simulink library "VAlib"  (Simulink 8.3)
settings: Solver=ode45  SolverMode=SingleTasking  StartTime=0.0  StopTime=10.0  RelTol=1e-3
undefined symbols (not defined in the file): automatic
libraries: VAlib x3, simulink x1
settings Model: Creator=aisakov  LastModifiedBy=lexx

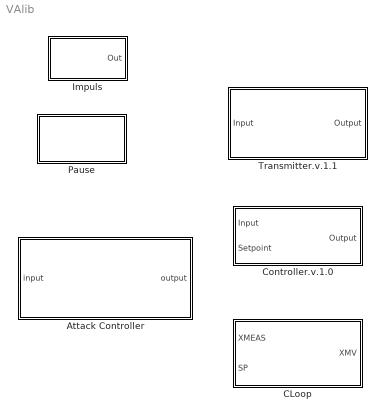
== system VAlib ==
  Attack Controller : Subsystem  mask(Attack controller){switch_mode=Integrity attack, atkMode=No attack, start=0, duration=1, Value=0, signalin=[], stime=-1, afterend=Holding final value}
      mask prompts: switch_mode "Attack Type:"; atkMode "Attack Mode:"; Value "Integrity Attack Value:"; signalin "Signal variable:"; stime "Sample time:"; afterend "Output after final:"
      mask help:
      | Attack controller block controls an attack on choosen variable on the specified time.
      | Attack types: DoS, Integrity and custom signal attack.
      | Modes: Step attack on specified time, Interval to specified time, Periodic and no attack.
      mask TypeOptions switch_mode: Integrity attack | DOS attack | Custom attack
      mask Callback switch_mode:
      | SM_MaskEnables = get_param(gcb, 'MaskEnables');
      | switch get_param(gcb, 'switch_mode')
      |     case 'Integrity attack'
      |         set_param([gcb,'/Switch value'], 'Value', '1');
      |         SM_MaskEnables{5} = 'on';
      |         SM_MaskEnables{6} = 'off';
      |         SM_MaskEnables{7} = 'off';
      |         SM_MaskEnables{8} = 'off';
      |     case 'DOS attack'
      |         set_param([gcb,'/Switch value'], 'Value', '3');
      |         SM_MaskEnables{5} = 'off';
      |         SM_MaskEnables{6} = 'off';
      |         SM_MaskEnables{7} = 'off';
      |         SM_MaskEnables{8} = 'off';
      |     case 'Custom attack'
      |         set_param([gcb,'/Switch value'], 'Value', '2');
      |         SM_MaskEnables{5} = 'off';
      |         SM_MaskEnables{6} = 'on';
      |         SM_MaskEnables{7} = 'on';
      |         SM_MaskEnables{8} = 'on';
      | end
      | set_param(gcb,'MaskEnables',SM_MaskEnables);
      | clear SM_MaskEnables;
      | 
      | % creat or remove block for custom attack
      | if strcmpi(get_param(gcb, 'switch_mode'), 'Custom attack') && ~exists_block([gcb '/SignalIn']) % creat block
      |     if exists_block([gcb, '/ReplaceBlock']);
      |         delete_line(gcb, 'ReplaceBlock/1', 'Multiport Switch/3');
      |         delete_block([gcb '/ReplaceBlock']);
      |     end
      | 
      |     add_block('built-in/FromWorkspace', [gcb '/SignalIn'], 'Position', [50 400 120 430]);
      |     add_line(gcb, 'SignalIn/1', 'Multiport Switch/3', 'autorouting', 'on');
      |     %set params
      |     set_param([gcb '/SignalIn'], 'SampleTime', '0');
      |     %set_param([gcb '/SignalIn'], 'VariableName', '[]');
      |     set_param([gcb '/SignalIn'], 'Interpolate', 'on');
      |     set_param([gcb '/SignalIn'], 'ZeroCross', 'off');
      |     %set_param([gcb '/' name], 'OutputAfterFinalValue', 'Setting to zero');
      |     %set_param([gcb '/' name], 'OutputAfterFinalValue', 'Cyclic repetition');
      |     %set_param([gcb '/' name], 'OutputAfterFinalValue', 'Extrapolation');
      |     %set_param([gcb '/' name], 'OutputAfterFinalValue', 'Holding final value');
      | 
      |     % forward signal parameters if set
      |     SW_signal = get_param(gcb, 'signalin');
      |     if strcmp(SW_signal, '[]') || strcmp(SW_signal, '') % signal not set
      |         set_param(gcb, 'signalin', '[]');
      |         set_param([gcb '/SignalIn'], 'VariableName', '[]');
      |         clear SW_signal;
      |         return;
      |     else    % signal set
      |         % check signal
      |         if ~exist(SW_signal)
      |             set_param(gcb, 'signalin', '[]');
      |             set_param([gcb '/SignalIn'], 'VariableName', '[]');
      |             warning(['Variable ' SW_signal ' not found.']);
      |             clear SW_signal;
      |             return;
      |         end
      |         SW_signal = evalin('base', SW_signal);
      |         if ~isvector(SW_signal)
      |             set_param(gcb, 'signalin', '');
      |             set_param([gcb '/SignalIn'], 'VariableName', '[]');
      |             warning(['Variable ' SW_signal ' must be a vector.']);
      |             clear SW_signal;
      |             return;
      |         end
      |         SW_stime = str2num(get_param(gcb, 'stime'));
      |         if isempty(SW_stime) || SW_stime < -1 || (SW_stime < 0 && SW_stime > -1)
      |             set_param(gcb, 'stime', '-1');
      |             SW_stime = -1;
      |             warning('Sample time must be a positive double or -1 for inherited value.');
      |         end
      | 
      |         if SW_stime == 0 || SW_stime == -1
      |             SW_stime = evalin('base', 'Ts_base');
      |         end
      | 
      |         SW_start = str2num(get_param(gcb, 'start'));
      |         SW_start = SW_stime * ceil(SW_start/SW_stime);
      |         signalstruct.time = SW_start:SW_stime:(SW_stime*(length(SW_signal) - 1) + SW_start);
      |         signalstruct.signals.values = SW_signal;
      | 
      | 		if strcmp(get_param(gcb, 'afterend'), 'Cyclic repetition')
      | 			SW_end = str2double(get_param(gcr, 'StopTime'));
      | 			while signalstruct.time(end) < SW_end
      | 				signalstruct.signals.values = [signalstruct.signals.values signalstruct.signals.values];
      | 				signalstruct.time = [signalstruct.time signalstruct.time+(signalstruct.time(end)-signalstruct.time(1))];
      | 			end
      | 		end
      | 
      | 		signalstruct.signals.values = signalstruct.signals.values(:);
      | 		signalstruct.time = signalstruct.time(:);
      |         %assignin('base', 'signalstruct', signalstruct)
      |         set_param([gcb '/SignalIn'], 'VariableName', 'signalstruct');
      |     end
      | 
      |     clear SW_signal;
      | 	clear SW_start;
      |     clear SW_stime;
      | 	clear SW_end;
      | elseif ~strcmpi(get_param(gcb, 'switch_mode'), 'Custom attack') && exists_block([gcb '/SignalIn']) % delete block
      |     delete_line(gcb, 'SignalIn/1', 'Multiport Switch/3');
      |     delete_block([gcb '/SignalIn']);
      |     % replace with constant value
      |     add_block(['built-in/Constant'], [gcb '/ReplaceBlock'], 'Position', [50 400 120 430]);
      |     add_line(gcb, ['ReplaceBlock/1'], 'Multiport Switch/3', 'autorouting', 'on');
      | end
      mask TypeOptions atkMode: Attack Type Controller/atkMode
      mask Callback atkMode:
      | AM_MaskEnables = get_param(gcb, 'MaskEnables');
      | switch get_param(gcb, 'atkMode');
      |     case 'No attack'
      |         AM_MaskEnables{3} = 'off';
      |         AM_MaskEnables{4} = 'off';
      |     case 'Step attack'
      |         AM_MaskEnables{3} = 'on';
      |         AM_MaskEnables{4} = 'off';
      |     otherwise
      |         AM_MaskEnables{3} = 'on';
      |         AM_MaskEnables{4} = 'on';
      | end
      | set_param(gcb, 'MaskEnables', AM_MaskEnables);
      | 
      | clear AM_MaskEnables;
      mask Callback start:
      | SS_start = get_param(gcb, 'start');
      | if strcmp(SS_start, '') % empty
      |     set_param(gcb, 'start', '0');
      |     SS_start = 0;
      | end
      | SS_start = str2num(SS_start);
      | if isempty(SS_start)
      |     set_param(gcb, 'start', '0');
      |     SS_start = 0;
      |     warning('Parameter value must be a nimeric value.');
      | end
      | 
      | % set to the subsystem
      | set_param([gcb '/Attack Type Controller'], 'start', get_param(gcb, 'start'));
      | 
      | % get correct signal parameters
      | if strcmpi(get_param(gcb, 'switch_mode'),'custom attack')
      |     if ~exists_block([gcb '/SignalIn'])
      |         clear SS_start;
      |         return
      |     end
      |     % forward signal parameters if set
      |     SS_signal = get_param(gcb, 'signalin');
      |     if strcmp(SS_signal, '[]') || strcmp(SS_signal, '') % signal not set
      |         clear SS_signal;
      |         clear SS_start;
      |         return;
      |     else    % signal set
      |         SS_signal = evalin('base', SS_signal);
      |         SS_stime = str2num(get_param(gcb, 'stime'));
      |         if isempty(SS_stime) || SS_stime < -1 || (SS_stime < 0 && SS_stime > -1)
      |             clear SS_signal;
      |             clear SS_start;
      |             set_param(gcb, 'stime', '-1');
      |             SS_stime = -1;
      |             warning('Sample time must be a positve double or -1 for inherited value.')
      |         end
      | 
      |         if SS_stime == 0 || SS_stime == -1
      |             SS_stime = evalin('base', 'Ts_base');
      |         end
      | 
      | 
      |         signalstruct.time = SS_start:SS_stime:(SS_stime*(length(SS_signal) - 1) + SS_start);
      |         signalstruct.signals.values = SS_signal;
      | 
      | 		if strcmp(get_param(gcb, 'afterend'), 'Cyclic repetition')
      | 			SS_end = str2double(get_param(gcr, 'StopTime'));
      | 			while signalstruct.time(end) < SS_end
      | 				signalstruct.signals.values = [signalstruct.signals.values signalstruct.signals.values];
      | 				signalstruct.time = [signalstruct.time signalstruct.time+(signalstruct.time(end)-signalstruct.time(1))];
      | 			end
      | 		end
      | 
      | 		signalstruct.signals.values = signalstruct.signals.values(:);
      | 		signalstruct.time = signalstruct.time(:);
      |         %assignin('base', 'signalstruct', signalstruct)
      |         set_param([gcb '/SignalIn'], 'VariableName', 'signalstruct');
      | 		clear SS_signal;
      | 		clear SS_start;
      | 		clear SS_stime;
      | 		clear SS_end;
      |     end
      | 
      | end
      mask TypeOptions duration: Attack Type Controller/duration
      mask TypeOptions Value: Integrity attack value/Value
      mask Callback signalin:
      | if ~exists_block([gcb '/SignalIn'])
      |     return;
      | end
      | 
      | % forward signal parameters if set
      | SI_signal = get_param(gcb, 'signalin');
      | if strcmp(SI_signal, '[]') || strcmp(SI_signal, '') % signal not set
      |     set_param([gcb '/SignalIn'], 'VariableName', '[]');
      |     set_param(gcb, 'signalin', '[]');
      |     clear SI_signal;
      | else
      |     if ~exist(SI_signal)
      |         set_param(gcb, 'signalin', '[]');
      |         set_param([gcb '/SignalIn'], 'VariableName', '[]');
      |         warning('VAC:AttackController:Signal variable', ['Variable ' SI_signal ' not found.']);
      |         clear SI_signal;
      |         return;
      |     end
      | 
      |     SI_signal = evalin('base', SI_signal);
      |     if ~isvector(SI_signal)
      |         set_param(gcb, 'signalin', '[]');
      |         set_param([gcb '/SignalIn'], 'VariableName', '[]');
      |         warning('VAC:AttackController:Signal variable', ['Variable ' SI_signal ' must be a vector.']);
      |         clear SI_signal;
      |         return;
      |     end
      | 
      |     SI_stime = str2num(get_param(gcb, 'stime'));
      |     if isempty(SI_stime) || SI_stime < -1 || (SI_stime < 0 && SI_stime > -1)
      |         set_param(gcb, 'stime', '-1');
      |         SI_stime = -1;
      |         warning('VAC:AttackController:Signal variable', 'Sample time must be a positive double or -1 for inherited value.');
      |     end
      | 
      |     if SI_stime == 0 || SI_stime == -1
      |         SI_stime = evalin('base', 'Ts_base');
      |     end
      | 
      | 	SI_start = str2double(get_param(gcb, 'start'));
      | 	SI_start = SI_stime * ceil(SI_start/SI_stime);
      | 	signalstruct.time = SI_start:SI_stime:(SI_stime*(length(SI_signal) - 1) + SI_start);
      | 	signalstruct.signals.values = SI_signal;
      | 
      |     if strcmp(get_param(gcb, 'afterend'), 'Cyclic repetition')
      | 		SI_end = str2double(get_param(gcr, 'StopTime'));
      | 		while signalstruct.time(end) < SI_end
      | 			signalstruct.signals.values = [signalstruct.signals.values signalstruct.signals.values];
      | 			signalstruct.time = [signalstruct.time signalstruct.time+(signalstruct.time(end)-signalstruct.time(1))];
      | 		end
      | 	end
      | 
      | 	signalstruct.signals.values = signalstruct.signals.values(:);
      | 	signalstruct.time = signalstruct.time(:);
      |     %assignin('base', 'signalstruct', signalstruct)
      |     set_param([gcb '/SignalIn'], 'VariableName', 'signalstruct');
      | 	clear SI_stime;
      | 	clear SI_start;
      | 	clear SI_signal;
      | 	clear SI_end;
      | end
      mask Callback stime:
      | SQ_stime = get_param(gcb, 'stime');
      | if strcmp(SQ_stime, '') % empty
      |     set_param(gcb, 'stime', '-1');
      |     SQ_stime = -1;
      | end
      | SQ_stime = str2num(SQ_stime);
      | if isempty(SQ_stime)
      |     set_param(gcb, 'stime', '-1');
      |     SQ_stime = -1;
      |     warning('VAC:AttackController:Sample time','Sample time must be a positve double or -1 for inherited value.')
      | end
      | 
      | % get correct signal parameters
      | if strcmpi(get_param(gcb, 'switch_mode'),'custom attack')
      |     if ~exists_block([gcb '/SignalIn'])
      |         clear SS_start;
      |         return
      |     end
      |     % forward signal parameters if set
      |     SQ_signal = get_param(gcb, 'signalin');
      |     if strcmp(SQ_signal, '[]') || strcmp(SQ_signal, '') % signal not set
      |         clear SQ_signal;
      |         clear SQ_stime;
      |         return;
      |     else    % signal set
      |         SQ_signal = evalin('base', SQ_signal);
      |         if SQ_stime == 0 || SQ_stime == -1
      |             SQ_stime = evalin('base', 'Ts_base');
      |         end
      | 
      | 		SQ_start = str2double(get_param(gcb, 'start'));
      | 		SQ_start = SQ_stime * ceil(SQ_start/SQ_stime);
      | 		signalstruct.time = SQ_start:SQ_stime:(SQ_stime*(length(SQ_signal) - 1) + SQ_start);
      |         signalstruct.signals.values = SQ_signal;
      | 
      | 		if strcmp(get_param(gcb, 'afterend'), 'Cyclic repetition')
      | 			SQ_end = str2double(get_param(gcr, 'StopTime'));
      | 			while signalstruct.time(end) < SQ_end
      | 				signalstruct.signals.values = [signalstruct.signals.values signalstruct.signals.values];
      | 				signalstruct.time = [signalstruct.time signalstruct.time+(signalstruct.time(end)-signalstruct.time(1))];
      | 			end
      | 		end
      | 
      | 		signalstruct.signals.values = signalstruct.signals.values(:);
      | 		signalstruct.time = signalstruct.time(:);
      |         %assignin('base', 'signalstruct', signalstruct)
      |         set_param([gcb '/SignalIn'], 'VariableName', 'signalstruct');
      |     end
      | 	clear SQ_signal;
      | 	clear SQ_start;
      | 	clear SQ_stime;
      | 	clear SQ_end;
      | end
      mask TypeOptions afterend: Extrapolation | Setting to zero | Holding final value | Cyclic repetition
      mask Callback afterend:
      | if ~exists_block([gcb '/SignalIn'])
      |     return
      | end
      | 
      | % forward choosen value
      | if ~strcmp(get_param(gcb, 'afterend'), 'Cyclic repetition')
      | 	set_param([gcb '/SignalIn'], 'OutputAfterFinalValue', get_param(gcb, 'afterend'));
      | end
      | 
      | % forward signal parameters if set
      | SA_signal = get_param(gcb, 'signalin');
      | if strcmp(SA_signal, '[]') || strcmp(SA_signal, '') % signal not set
      |     set_param([gcb '/SignalIn'], 'VariableName', '[]');
      |     set_param(gcb, 'signalin', '[]');
      |     clear SA_signal;
      | else
      |     if ~exist(SA_signal)
      |         set_param(gcb, 'signalin', '[]');
      |         set_param([gcb '/SignalIn'], 'VariableName', '[]');
      |         warning('VAC:AttackController:After end', ['Variable ' SA_signal ' not found.']);
      |         clear SA_signal;
      |         return;
      |     end
      | 
      |     SA_signal = evalin('base', SA_signal);
      |     if ~isvector(SA_signal)
      |         set_param(gcb, 'signalin', '[]');
      |         set_param([gcb '/SignalIn'], 'VariableName', '[]');
      |         warning('VAC:AttackController:After end', ['Variable ' SA_signal ' must be a vector.']);
      |         clear SA_signal;
      |         return;
      |     end
      | 
      |     SA_stime = str2num(get_param(gcb, 'stime'));
      |     if isempty(SA_stime) || SA_stime < -1 || (SA_stime < 0 && SA_stime > -1)
      |         set_param(gcb, 'stime', '-1');
      |         SA_stime = -1;
      |         warning('VAC:AttackController:After end', 'Sample time must be a positive double or -1 for inherited value.');
      |     end
      | 
      |     if SA_stime == 0 || SA_stime == -1
      |         SA_stime = evalin('base', 'Ts_base');
      |     end
      | 
      | 	SA_start = str2double(get_param(gcb, 'start'));
      | 	SA_start = SA_stime * ceil(SA_start/SA_stime);
      | 	signalstruct.time = SA_start:SA_stime:(SA_stime*(length(SA_signal) - 1) + SA_start);
      | 	signalstruct.signals.values = SA_signal;
      | 
      | 	if strcmp(get_param(gcb, 'afterend'), 'Cyclic repetition')
      | 		SA_end = str2double(get_param(gcr, 'StopTime'));
      | 		while signalstruct.time(end) < SA_end
      | 			signalstruct.signals.values = [signalstruct.signals.values signalstruct.signals.values];
      | 			signalstruct.time = [signalstruct.time signalstruct.time+(signalstruct.time(end)-signalstruct.time(1))];
      | 		end
      |     end
      | 
      |     signalstruct.time = signalstruct.time(:);
      | 	signalstruct.signals.values = signalstruct.signals.values(:);
      |     %assignin('base', 'signalstruct', signalstruct)
      |     set_param([gcb '/SignalIn'], 'VariableName', 'signalstruct');
      | 
      | 	clear SA_stime;
      | 	clear SA_start;
      | 	clear SA_signal;
      | 	clear SA_end;
      | end
      mask Display:
      | disp([get_param(gcb, 'switch_mode') '\n' get_param(gcb, 'atkMode')])
      | port_label('input', 1, 'signal in')
      | port_label('output', 1, 'signal out')
  CLoop : Subsystem  mask{ctype=1 (Proportional only), mode=1 (automatic), gain=1, reset=1, csampling=1, lowmeas=1, highmeas=2, lowmv=1, highmv=2, deadtime=1, tau=1, tsampling=1, x0mv=1, x0xs=1, x0sp=1}
      mask prompts: ctype "Type:"; reset "Reset time: (in minutes)"; csampling "Sampling time: (in minutes)"; lowmeas "Low limit of measurement:"; highmeas "High limit of measurement:"; lowmv "Low limit of MV:"; highmv "High limit of MV:"; deadtime "Dead time: (in minutes)"; tau "Lag time: (in minutes)"; tsampling "Sampling time: (in minutes)"; x0mv "MV:"; x0xs "XS:"; x0sp "SP:"
      mask TypeOptions ctype: Controller/ctype
      mask TypeOptions mode: Controller/mode
      mask TypeOptions gain: Gain/Value
      mask TypeOptions reset: Reset/Value
      mask TypeOptions csampling: Sampling/Value
      mask TypeOptions lowmeas: LowLimitMeas/Value
      mask TypeOptions highmeas: HighLimitMeas/Value
      mask TypeOptions lowmv: LowLimitMv/Value
      mask TypeOptions highmv: HighLimitMv/Value
      mask DialogControl Container8 Prompt: Parameters
      mask DialogControl Container18 Prompt: Parameters
      mask DialogControl Container16 Prompt: Parameters
      mask Display:
      | disp([ControllerType.FromValue(ctype).String '-Controller' ...
      |     '\nGain:' num2str(gain) ...
      |     '\nReset time:' num2str(reset)])
      | port_label('output', 1, 'OUT')
      | port_label('input', 1, 'IN')
      | port_label('input', 2, 'SP')
  Controller.v.1.0 : Subsystem  mask{ctype=0 (PI), mode=1 (automatic), pgain=1, gain=1, reset=1, sampling=1, lowmeas=1, highmeas=1, lowmv=1, highmv=1, mvx0=0, xix0=0}
      mask prompts: ctype "Type:"; pgain "Process gain: (1 for positive gain, -1 for negative gain)"; reset "Reset time: (in minute)"; sampling "Sampling time: (in minute)"; lowmeas "Low limit of measurement:"; highmeas "High limit of measurement:"; lowmv "Low limit of MV:"; highmv "High limit of MV:"; mvx0 "MV"; xix0 "XI"
      mask TypeOptions ctype: 0 (PI) | 1 (Proportional only) | 2 (Fixed)
      mask TypeOptions mode: 1 (automatic) | 2 (manual) | 3 (autotune)
      mask TypeOptions pgain: GainSign/Value
      mask TypeOptions gain: Gain/Value
      mask TypeOptions reset: Reset/Value
      mask TypeOptions sampling: Sampling/Value
      mask TypeOptions lowmeas: LowLimitMeas/Value
      mask TypeOptions highmeas: HighLimitMeas/Value
      mask TypeOptions lowmv: LowLimitMv/Value
      mask TypeOptions highmv: HighLimitMv/Value
      mask TypeOptions mvx0: MV Memory/X0
      mask TypeOptions xix0: XI Memory/X0
      mask Display:
      | fprintf('Controller')
      | port_label('output', 1, 'OUT')
      | port_label('input', 1, 'IN')
      | port_label('input', 2, 'SP')
  Impuls : Subsystem  mask{amplitude=1, duration=5, delay=1}
      mask prompts: duration "Pulse width:"; delay "Pulse delay:"
      mask Display:
      | x = [0 1 1 2 2 3];
      | y = [0 0 1 1 0 0];
      | plot(x,y)
  Pause : Subsystem  mask(Pause){Value=-1}
      mask help: Make a pause at spiecified time
      mask TypeOptions Value: Constant/Value
      mask Display:
      | patch([0 7], [0 5], [1 1 1])
      | patch([2 3 3 2 2], [4 4 1 1 4],[0 0 0])
      | patch([4 5 5 4 4], [4 4 1 1 4],[0 0 0])
  Transmitter.v.1.1 : Subsystem  mask{deadtime=1, tau=1, sampling=1, lowmeas=1, highmeas=1, xxx0=0, yyy0=0}
      mask prompts: deadtime "Dead time:"; tau "Lag:"; sampling "Sampling time:"; lowmeas "Low limit of measurement:"; highmeas "High limit of measurement:"; xxx0 "XXX:"; yyy0 "YYY:"
      mask TypeOptions deadtime: DeadTime/Value
      mask TypeOptions tau: Lag/Value
      mask TypeOptions sampling: SamplingTime/Value
      mask TypeOptions lowmeas: LowMeas/Value
      mask TypeOptions highmeas: HighMeas/Value
      mask TypeOptions xxx0: XXX Initial/X0
      mask TypeOptions yyy0: YYY Initial/X0
      mask Display:
      | fprintf('Transmitter')
      | port_label('output', 1, 'OUT')
      | port_label('input', 1, 'IN')

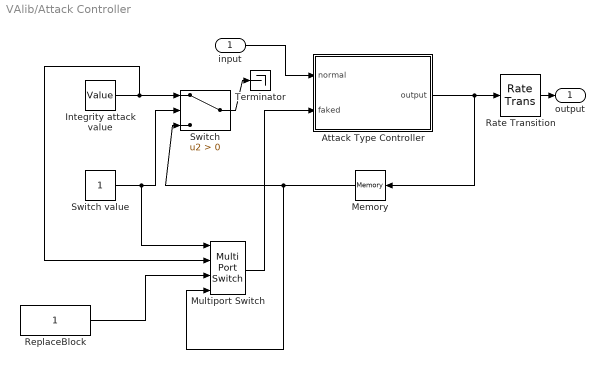
== system VAlib/Attack Controller ==
  input : Inport
  Attack Type Controller : Subsystem  Variant=on  OverrideUsingVariant=normal_forward_controller  mask{atkMode=No attack, start=0, duration=duration}
      mask prompts: atkMode "Attack Mode:"
      mask TypeOptions atkMode: No attack | Step attack | Interval attack | Periodical attack
      mask Callback atkMode:
      | switch get_param(gcb,'atkMode');
      |     case 'Step attack'
      |         set_param(gcb, 'OverrideUsingVariant', 'step_forward_controller');
      |     case 'Interval attack'
      |         set_param(gcb, 'OverrideUsingVariant', 'interval_forward_controller');
      |     case 'Periodical attack'
      |         set_param(gcb, 'OverrideUsingVariant', 'periodical_forward_controller');
      |     otherwise
      |         set_param(gcb, 'OverrideUsingVariant', 'normal_forward_controller');
      | end
      mask Display: eval(get_param([gcb '/' strrep(get_param(gcb, 'ActiveVariant'), '_', ' ')], 'MaskDisplay'));
  Integrity attack value : Constant  Value=Value
  Memory : Memory
  Multiport Switch : MultiPortSwitch
  Rate Transition : RateTransition  Deterministic=off
  ReplaceBlock : Constant
  Switch : Switch  Criteria=u2 > Threshold
  Switch value : Constant
  Terminator : Terminator
  output : Outport
  wires:
  Integrity attack value/1 -> Multiport Switch/2, Switch/1
  Switch value/1 -> Multiport Switch/1, Switch/2
  input/1 -> Attack Type Controller/1(normal)
  Memory/1 -> Multiport Switch/4, Switch/3
  Multiport Switch/1 -> Attack Type Controller/2(faked)
  Switch/1 -> Terminator/1
  ReplaceBlock/1 -> Multiport Switch/3
  Attack Type Controller/1(output) -> Rate Transition/1, Memory/1
  Rate Transition/1 -> output/1

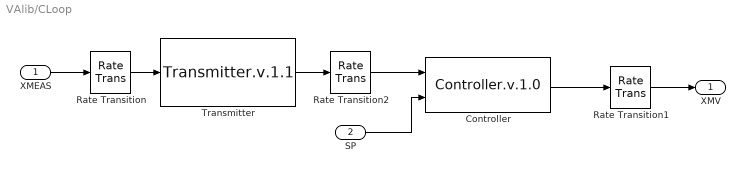
== system VAlib/CLoop ==
  XMEAS : Inport
  SP : Inport  Port=2
  Controller : VAlib/Controller.v.1.0  ctype=1 (Proportional only)  mode=1 (automatic)  pgain=sign(gain)  gain=abs(gain)  reset=reset  sampling=1/csampling  lowmeas=lowmeas  highmeas=highmeas  lowmv=lowmv  highmv=highmv  mvx0=x0mv  xix0=(x0mv - lowmv)/(highmv-lowmv)-gain*((x0sp-lowmeas)/(highmeas-lowmeas)-(x0xs-lowmeas)/(highmeas-lowmeas))
  Rate Transition : RateTransition  Deterministic=off  X0=x0xs  OutPortSampleTime=1/(tsampling*60)
  Rate Transition1 : RateTransition  Deterministic=off  X0=x0mv
  Rate Transition2 : RateTransition  Deterministic=off  X0=(x0xs-lowmeas)/(highmeas-lowmeas)  OutPortSampleTime=1/(csampling*60)
  Transmitter : VAlib/Transmitter.v.1.1  deadtime=deadtime  tau=tau  sampling=1/tsampling  lowmeas=lowmeas  highmeas=highmeas  xxx0=ones(1, 1+deadtime*tsampling) * ((x0xs-lowmeas)/(highmeas-lowmeas))  yyy0=(x0xs-lowmeas)/(highmeas-lowmeas)
  XMV : Outport
  wires:
  SP/1 -> Controller/2
  Rate Transition/1 -> Transmitter/1
  XMEAS/1 -> Rate Transition/1
  Rate Transition2/1 -> Controller/1
  Rate Transition1/1 -> XMV/1
  Transmitter/1 -> Rate Transition2/1
  Controller/1 -> Rate Transition1/1

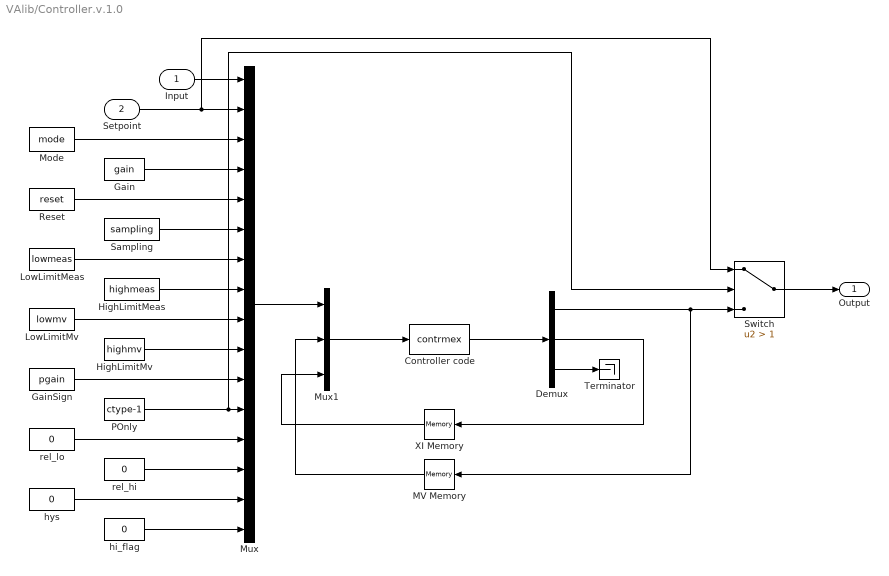
== system VAlib/Controller.v.1.0 ==
  Input : Inport
  Setpoint : Inport  Port=2
  Controller code : S-Function  FunctionName=contrmex  Parameters=[sampling]  EnableBusSupport=off
  Demux : Demux  Outputs=3
  Gain : Constant  Value=gain
  GainSign : Constant  Value=pgain
  HighLimitMeas : Constant  Value=highmeas
  HighLimitMv : Constant  Value=highmv
  LowLimitMeas : Constant  Value=lowmeas
  LowLimitMv : Constant  Value=lowmv
  MV Memory : Memory  X0=mvx0  InheritSampleTime=on  LinearizeMemory=on
  Mode : Constant  Value=mode
  Mux : Mux  Inputs=16
  Mux1 : Mux  Inputs=3
  POnly : Constant  Value=ctype-1
  Reset : Constant  Value=reset
  Sampling : Constant  Value=sampling
  Switch : Switch  Criteria=u2 > Threshold  Threshold=1
  Terminator : Terminator
  XI Memory : Memory  X0=xix0  InheritSampleTime=on  LinearizeMemory=on
  hi_flag : Constant  Value=0
  hys : Constant  Value=0
  rel_hi : Constant  Value=0
  rel_lo : Constant  Value=0
  Output : Outport
  wires:
  XI Memory/1 -> Mux1/3
  Input/1 -> Mux/1
  Setpoint/1 -> Switch/1, Mux/2
  Mux/1 -> Mux1/1
  Mode/1 -> Mux/3
  Gain/1 -> Mux/4
  Reset/1 -> Mux/5
  Sampling/1 -> Mux/6
  LowLimitMeas/1 -> Mux/7
  HighLimitMeas/1 -> Mux/8
  LowLimitMv/1 -> Mux/9
  HighLimitMv/1 -> Mux/10
  GainSign/1 -> Mux/11
  POnly/1 -> Switch/2, Mux/12
  rel_lo/1 -> Mux/13
  rel_hi/1 -> Mux/14
  hys/1 -> Mux/15
  hi_flag/1 -> Mux/16
  Demux/1 -> Switch/3, MV Memory/1
  MV Memory/1 -> Mux1/2
  Demux/3 -> Terminator/1
  Demux/2 -> XI Memory/1
  Mux1/1 -> Controller code/1
  Controller code/1 -> Demux/1
  Switch/1 -> Output/1

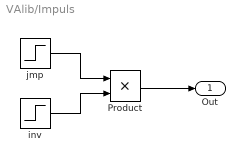
== system VAlib/Impuls ==
  Product : Product
  inv : Step  Time=delay + duration  Before=amplitude  After=0  SampleTime=0
  jmp : Step  Time=delay  After=amplitude  SampleTime=0
  Out : Outport
  wires:
  jmp/1 -> Product/1
  inv/1 -> Product/2
  Product/1 -> Out/1

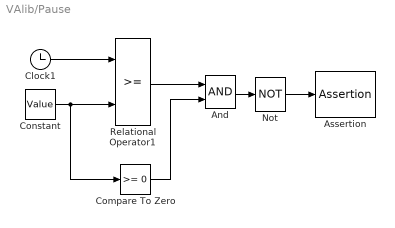
== system VAlib/Pause ==
  And : Logic  AllPortsSameDT=off  OutDataTypeStr=boolean
  Assertion : Assertion  AssertionFailFcn=|  StopWhenAssertionFail=off
      | set_param(bdroot,'SimulationCommand','pause'),
      | disp(sprintf('\nSimulation paused.'))
  Clock1 : Clock
  Compare To Zero : simulink/Logic and Bit Operations/Compare To Zero  relop=>=  OutDataTypeStr=boolean
  Constant : Constant  Value=Value
  Not : Logic  Operator=NOT  AllPortsSameDT=off  OutDataTypeStr=boolean
  Relational Operator1 : RelationalOperator  OutDataTypeStr=boolean
  wires:
  Clock1/1 -> Relational Operator1/1
  Relational Operator1/1 -> And/1
  Constant/1 -> Compare To Zero/1, Relational Operator1/2
  And/1 -> Not/1
  Compare To Zero/1 -> And/2
  Not/1 -> Assertion/1

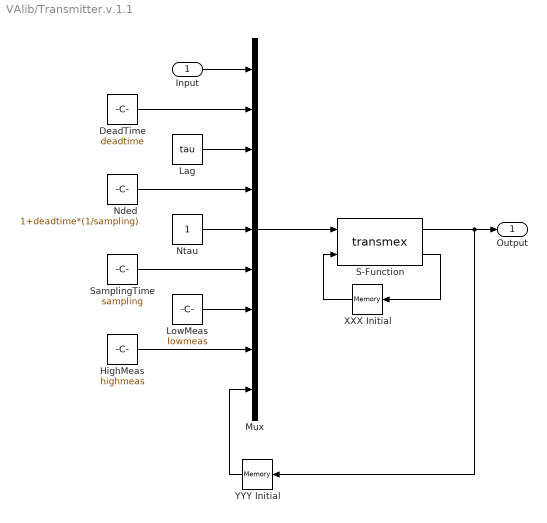
== system VAlib/Transmitter.v.1.1 ==
  Input : Inport
  DeadTime : Constant  Value=deadtime
  HighMeas : Constant  Value=highmeas
  Lag : Constant  Value=tau
  LowMeas : Constant  Value=lowmeas
  Mux : Mux  Inputs=9
  Nded : Constant  Value=1+deadtime*(1/sampling)
  Ntau : Constant
  S-Function : S-Function  FunctionName=transmex  Parameters=[sampling]  EnableBusSupport=off
  SamplingTime : Constant  Value=sampling
  XXX Initial : Memory  X0=xxx0  InheritSampleTime=on  LinearizeMemory=on
  YYY Initial : Memory  X0=yyy0  InheritSampleTime=on  LinearizeMemory=on
  Output : Outport
  wires:
  Input/1 -> Mux/1
  S-Function/1 -> YYY Initial/1, Output/1
  S-Function/2 -> XXX Initial/1
  XXX Initial/1 -> S-Function/2
  YYY Initial/1 -> Mux/9
  DeadTime/1 -> Mux/2
  Lag/1 -> Mux/3
  Nded/1 -> Mux/4
  Ntau/1 -> Mux/5
  SamplingTime/1 -> Mux/6
  LowMeas/1 -> Mux/7
  HighMeas/1 -> Mux/8
  Mux/1 -> S-Function/1

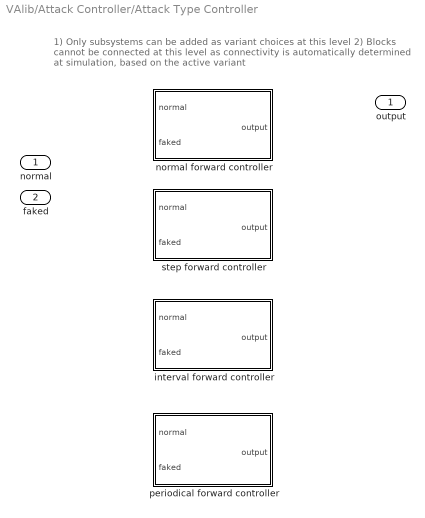
== system VAlib/Attack Controller/Attack Type Controller ==
  note: 1) Only subsystems can be added as variant choices at this level
      | 2) Blocks cannot be connected at this level as connectivity is
      | automatically determined at simulation, based on the active variant
  normal : Inport
  faked : Inport  Port=2
  interval forward controller : Subsystem  VariantControl=interval_forward_controller
      mask Display:
      | disp('IFC')
      | port_label('input', 1, 'normal in')
      | port_label('input', 2, 'faked in')
      | port_label('output', 1, 'out')
  normal forward controller : Subsystem  VariantControl=normal_forward_controller
      mask Display:
      | disp('NFC')
      | port_label('input', 1, 'normal in')
      | port_label('input', 2, 'faked in')
      | port_label('output', 1, 'out')
  periodical forward controller : Subsystem  VariantControl=periodical_forward_controller
      mask Display:
      | disp('PFC')
      | port_label('input', 1, 'normal in')
      | port_label('input', 2, 'faked in')
      | port_label('output', 1, 'out')
  step forward controller : Subsystem  VariantControl=step_forward_controller
      mask Display:
      | disp('SFC')
      | port_label('input', 1, 'normal in')
      | port_label('input', 2, 'faked in')
      | port_label('output', 1, 'out')
  output : Outport

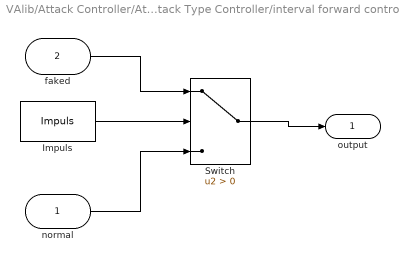
== system VAlib/Attack Controller/Attack Type Controller/interval forward controller ==
  normal : Inport
  faked : Inport  Port=2
  Impuls : VAlib/Impuls  amplitude=1  duration=duration  delay=start
  Switch : Switch  Criteria=u2 > Threshold
  output : Outport
  wires:
  faked/1 -> Switch/1
  normal/1 -> Switch/3
  Impuls/1 -> Switch/2
  Switch/1 -> output/1

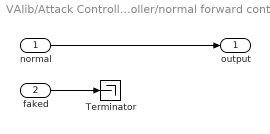
== system VAlib/Attack Controller/Attack Type Controller/normal forward controller ==
  normal : Inport
  faked : Inport  Port=2
  Terminator : Terminator
  output : Outport
  wires:
  normal/1 -> output/1
  faked/1 -> Terminator/1

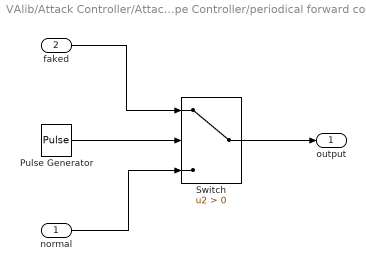
== system VAlib/Attack Controller/Attack Type Controller/periodical forward controller ==
  normal : Inport
  faked : Inport  Port=2
  Pulse Generator : DiscretePulseGenerator  PulseType=Time based  Period=duration + start  PulseWidth=100*duration/(duration + start)  PhaseDelay=start
  Switch : Switch  Criteria=u2 > Threshold
  output : Outport
  wires:
  faked/1 -> Switch/1
  normal/1 -> Switch/3
  Pulse Generator/1 -> Switch/2
  Switch/1 -> output/1

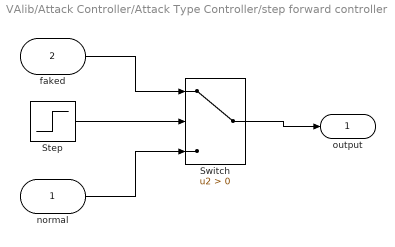
== system VAlib/Attack Controller/Attack Type Controller/step forward controller ==
  normal : Inport
  faked : Inport  Port=2
  Step : Step  Time=start  SampleTime=0
  Switch : Switch  Criteria=u2 > Threshold
  output : Outport
  wires:
  faked/1 -> Switch/1
  normal/1 -> Switch/3
  Step/1 -> Switch/2
  Switch/1 -> output/1
